simulink model "gm_sampleModel1541_4_sub_sub_sub"  (R2023a)
settings: Solver=VariableStepAuto  StartTime=0.0  StopTime=10.0  RelTol=1e-3
libraries: hdlsllib x4, simulink x3
settings Model: Creator=user1  LastModifiedBy=user1
settings OptimizationCC: BlockReduction=off  ConditionallyExecuteInputs=off
settings DebuggingCC: InheritedTsInSrcMsg=none

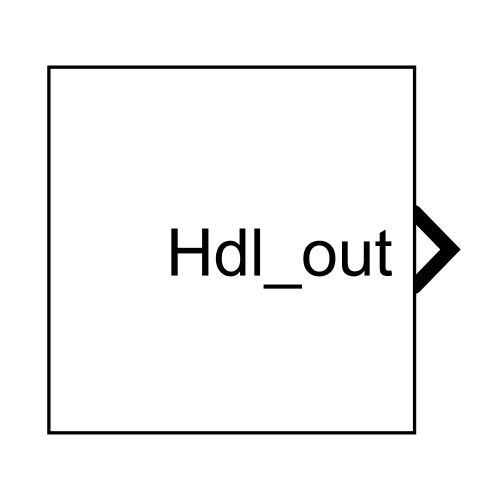
[thumbnail: Simulink's stored preview of the top-level diagram]
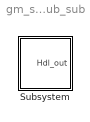
== system gm_sampleModel1541_4_sub_sub_sub ==
  Subsystem : Subsystem

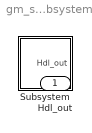
== system gm_sampleModel1541_4_sub_sub_sub/Subsystem ==
  Subsystem : Subsystem
  Hdl_out : Outport  OutDataTypeStr=uint8

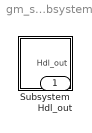
== system gm_sampleModel1541_4_sub_sub_sub/Subsystem/Subsystem ==
  Subsystem : Subsystem
  Hdl_out : Outport  OutDataTypeStr=uint8

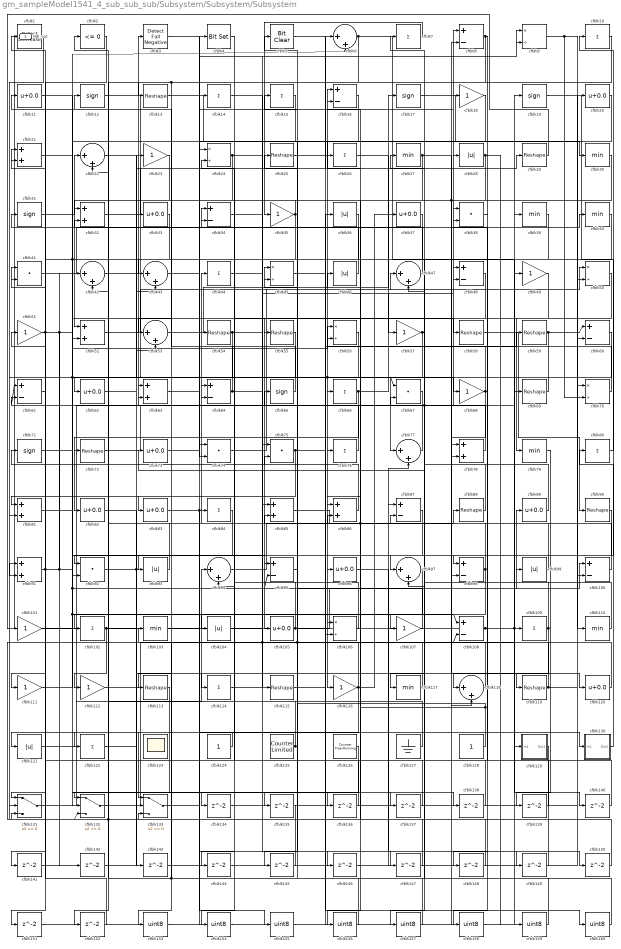
== system gm_sampleModel1541_4_sub_sub_sub/Subsystem/Subsystem/Subsystem ==
  cfblk1 : simulink/Logic and Bit Operations/Detect Decrease  vinit=0.0  OutDataTypeStr=uint8
      settings: LibrarySourceBlock=|
      | hdlsllib/Logic and Bit
      | Operations/Detect
      | Decrease
  cfblk{7,10,14..15,26,44,66,76,80,84,102,109,114,122} (14 alike) : Sum  Inputs=+  OutDataTypeStr=uint8
  cfblk{8,16,34,48,60..61,64,87,95,98,100,108} (12 alike) : Sum  Inputs=+-  OutDataTypeStr=uint8
  cfblk{18,23,35,49,51,57,68,101,107,111..112,116} (12 alike) : Gain  OutDataTypeStr=uint8
  cfblk{27,30,39..40,79,103,110,117} (8 alike) : MinMax  OutDataTypeStr=uint8
  cfblk{28,36,46,93,99,104,121} (7 alike) : Abs  OutDataTypeStr=uint8  SaturateOnIntegerOverflow=off
  cfblk{11,20,33,37,62,73,82..83,89,96,105,120} (12 alike) : Bias  Bias=0.0  SaturateOnIntegerOverflow=off
  cfblk{9,24,45,50,56,70,106} (7 alike) : Product  Inputs=*/  OutDataTypeStr=uint8  RndMeth=Zero  SaturateOnIntegerOverflow=on
  cfblk{13,25,29,54..55,58..59,69,72,88,90,113,115,119} (14 alike) : Reshape
  cfblk{6,22,42..43,47,53,77,94,97,118} (10 alike) : Sum  Inputs=|++  OutDataTypeStr=uint8
  cfblk{12,17,19,31,65,71} (6 alike) : Signum
  cfblk123 : Scope
      settings: Floating=on
  cfblk124 : Constant  OutDataTypeStr=uint8  SampleTime=-1
  cfblk125 : hdlsllib/Sources/Counter Limited  uplimit=7  tsamp=-1
  cfblk126 : hdlsllib/Sources/Counter Free-Running  NumBits=16  tsamp=-1
  cfblk127 : Ground
  cfblk128 : Constant  OutDataTypeStr=uint8  SampleTime=-1
  cfblk129 : Subsystem
      settings: LibrarySourceBlock=|
      | hdlsllib/Ports &
      | Subsystems/Subsystem
  cfblk130 : Subsystem
      settings: LibrarySourceBlock=|
      | hdlsllib/Ports &
      | Subsystems/Subsystem
  cfblk131 : Switch  OutDataTypeStr=uint8  SaturateOnIntegerOverflow=off  InputSameDT=off
  cfblk132 : Switch  OutDataTypeStr=uint8  SaturateOnIntegerOverflow=off  InputSameDT=off
  cfblk133 : Switch  OutDataTypeStr=uint8  SaturateOnIntegerOverflow=off  InputSameDT=off
  cfblk{134..152} (19 alike) : Delay  SampleTime=1
  cfblk{153..160} (8 alike) : DataTypeConversion  OutDataTypeStr=uint8  SaturateOnIntegerOverflow=off  RndMeth=Floor
  cfblk2 : hdlsllib/Logic and Bit Operations/Compare To Zero  relop=<=  OutDataTypeStr=uint8
  cfblk{21,32,52,63,78,81,85..86,91} (9 alike) : Sum  OutDataTypeStr=uint8
  cfblk3 : hdlsllib/Logic and Bit Operations/Detect Fall Negative  vinit=0  OutDataTypeStr=uint8
  cfblk{38,41,67,74..75,92} (6 alike) : DotProduct  OutDataTypeStr=uint8
  cfblk4 : simulink/Logic and Bit Operations/Bit Set  iBit=0
      settings: LibrarySourceBlock=|
      | hdlsllib/Logic and Bit
      | Operations/Bit Set
  cfblk5 : simulink/Logic and Bit Operations/Bit Clear  iBit=0
      settings: LibrarySourceBlock=|
      | hdlsllib/Logic and Bit
      | Operations/Bit Clear
  Hdl_out : Outport  OutDataTypeStr=uint8
  wires:
  cfblk160/1 -> cfblk97/2
  cfblk5/1 -> cfblk160/1
  cfblk159/1 -> cfblk5/1
  cfblk158/1 -> cfblk39/1
  cfblk157/1 -> cfblk132/3, cfblk12/1, cfblk133/3
  cfblk156/1 -> cfblk103/1
  cfblk30/1 -> cfblk156/1
  cfblk155/1 -> cfblk36/1
  cfblk103/1 -> cfblk155/1
  cfblk154/1 -> cfblk109/1
  cfblk4/1 -> cfblk154/1
  cfblk153/1 -> cfblk4/1
  cfblk152/1 -> cfblk41/2
  cfblk90/1 -> cfblk152/1
  cfblk151/1 -> cfblk118/2
  cfblk150/1 -> cfblk78/1
  cfblk44/1 -> cfblk150/1
  cfblk149/1 -> cfblk131/2
  cfblk96/1 -> cfblk149/1
  cfblk148/1 -> cfblk86/2
  cfblk147/1 -> cfblk74/1
  cfblk45/1 -> cfblk147/1
  cfblk146/1 -> cfblk8/2
  cfblk133/1 -> cfblk146/1
  cfblk145/1 -> cfblk91/1
  cfblk16/1 -> cfblk145/1
  cfblk144/1 -> cfblk100/2
  cfblk48/1 -> cfblk144/1
  cfblk143/1 -> cfblk77/2
  cfblk82/1 -> cfblk143/1
  cfblk142/1 -> cfblk70/1
  cfblk141/1 -> cfblk43/2
  cfblk140/1 -> cfblk38/2
  cfblk139/1 -> cfblk87/1
  cfblk79/1 -> cfblk139/1
  cfblk138/1 -> cfblk47/2
  cfblk137/1 -> cfblk1/1
  cfblk14/1 -> cfblk137/1
  cfblk136/1 -> cfblk64/2
  cfblk135/1 -> cfblk131/3
  cfblk60/1 -> cfblk135/1
  cfblk134/1 -> cfblk50/2
  cfblk97/1 -> cfblk134/1
  cfblk26/1 -> cfblk57/1
  cfblk33/1 -> cfblk81/1
  cfblk113/1 -> cfblk132/2
  cfblk46/1 -> cfblk24/2
  cfblk24/1 -> cfblk113/1, cfblk136/1
  cfblk100/1 -> cfblk26/1, cfblk42/2
  cfblk88/1 -> cfblk33/1, cfblk61/1
  cfblk20/1 -> cfblk92/2
  cfblk120/1 -> cfblk7/1
  cfblk81/1 -> cfblk106/1
  cfblk61/1 -> cfblk21/1
  cfblk127/1 -> cfblk22/2
  cfblk117/1 -> cfblk75/2
  cfblk114/1 -> cfblk46/1, cfblk108/2
  cfblk126/1 -> cfblk132/1
  cfblk89/1 -> cfblk31/1
  cfblk47/1 -> cfblk34/2
  cfblk10/1 -> cfblk13/1
  cfblk77/1 -> cfblk64/1
  cfblk1/1 -> cfblk91/2
  cfblk106/1 -> cfblk71/1
  cfblk116/1 -> cfblk45/1, cfblk37/1, cfblk133/1
  cfblk109/1 -> cfblk73/1, cfblk148/1
  cfblk107/1 -> cfblk25/1
  cfblk63/1 -> cfblk14/1
  cfblk95/1 -> cfblk65/1
  cfblk15/1 -> cfblk74/2
  cfblk9/1 -> cfblk60/2, cfblk70/2
  cfblk36/1 -> cfblk43/1
  cfblk13/1 -> cfblk75/1
  cfblk62/1 -> cfblk29/1
  cfblk87/1 -> cfblk92/1
  cfblk43/1 -> cfblk9/1
  cfblk132/1 -> cfblk69/1
  cfblk83/1 -> cfblk18/1, cfblk130/1(In1)
  cfblk68/1 -> cfblk16/2, cfblk98/2, cfblk158/1
  cfblk21/1 -> cfblk66/1, cfblk67/1, cfblk107/1
  cfblk128/1 -> cfblk85/2, cfblk56/2
  cfblk66/1 -> cfblk82/1, cfblk48/2
  cfblk85/1 -> cfblk87/2
  cfblk112/1 -> cfblk120/1
  cfblk72/1 -> cfblk19/1
  cfblk22/1 -> cfblk68/1
  cfblk91/1 -> cfblk95/1, cfblk42/1, cfblk41/1
  cfblk92/1 -> cfblk114/1, cfblk67/2
  cfblk59/1 -> cfblk60/1, cfblk81/2
  cfblk73/1 -> cfblk24/1
  cfblk98/1 -> cfblk122/1, cfblk27/1
  cfblk51/1 -> cfblk133/2, cfblk142/1, cfblk21/2
  cfblk111/1 -> cfblk6/2, cfblk95/2
  cfblk2/1 -> cfblk111/1
  cfblk130/1(Out1) -> cfblk80/1
  cfblk32/1 -> cfblk6/1
  cfblk11/1 -> cfblk55/1
  cfblk84/1 -> cfblk93/1
  cfblk101/1 -> cfblk56/1
  cfblk57/1 -> cfblk77/1, cfblk117/1
  cfblk31/1 -> cfblk22/1
  cfblk65/1 -> cfblk34/1
  cfblk55/1 -> cfblk131/1
  cfblk67/1 -> cfblk63/2
  cfblk8/1 -> cfblk102/1, cfblk83/1, cfblk98/1
  cfblk119/1 -> cfblk20/1, cfblk94/2
  cfblk40/1 -> cfblk104/1
  cfblk17/1 -> cfblk110/1
  cfblk115/1 -> cfblk59/1
  cfblk71/1 -> cfblk108/1, cfblk138/1
  cfblk86/1 -> cfblk54/1
  cfblk80/1 -> cfblk10/1
  cfblk125/1 -> cfblk84/1, cfblk45/2
  cfblk108/1 -> cfblk49/1, cfblk140/1, Hdl_out/1
  cfblk35/1 -> cfblk52/2, cfblk141/1, cfblk32/1
  cfblk122/1 -> cfblk23/1
  cfblk37/1 -> cfblk86/1
  cfblk23/1 -> cfblk52/1
  cfblk105/1 -> cfblk100/1, cfblk32/2
  cfblk93/1 -> cfblk2/1
  cfblk53/1 -> cfblk17/1
  cfblk129/1(Out1) -> cfblk51/1
  cfblk75/1 -> cfblk40/1, cfblk151/1
  cfblk121/1 -> cfblk94/1
  cfblk102/1 -> cfblk112/1, cfblk53/2
  cfblk12/1 -> cfblk115/1
  cfblk3/1 -> cfblk30/1
  cfblk76/1 -> cfblk63/1
  cfblk74/1 -> cfblk50/1
  cfblk29/1 -> cfblk101/1
  cfblk54/1 -> cfblk48/1, cfblk153/1
  cfblk58/1 -> cfblk90/1
  cfblk41/1 -> cfblk38/1
  cfblk38/1 -> cfblk118/1
  cfblk28/1 -> cfblk72/1, cfblk78/2, cfblk159/1
  cfblk6/1 -> cfblk129/1(In1), cfblk53/1
  cfblk42/1 -> cfblk58/1
  cfblk25/1 -> cfblk16/1
  cfblk64/1 -> cfblk11/1, cfblk9/2
  cfblk39/1 -> cfblk157/1
  cfblk118/1 -> cfblk15/1, cfblk61/2
  cfblk34/1 -> cfblk85/1
  cfblk49/1 -> cfblk79/1
  cfblk104/1 -> cfblk99/1
  cfblk131/1 -> cfblk28/1
  cfblk94/1 -> cfblk88/1
  cfblk78/1 -> cfblk3/1
  cfblk70/1 -> cfblk8/1
  cfblk7/1 -> cfblk35/1
  cfblk52/1 -> cfblk47/1
  cfblk56/1 -> cfblk76/1, cfblk106/2
  cfblk124/1 -> cfblk121/1
  cfblk18/1 -> cfblk96/1
  cfblk27/1 -> cfblk116/1, cfblk119/1
  cfblk99/1 -> cfblk44/1
  cfblk110/1 -> cfblk89/1
  cfblk69/1 -> cfblk62/1
  cfblk19/1 -> cfblk97/1
  cfblk50/1 -> cfblk105/1

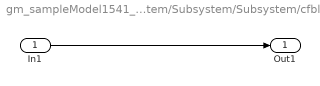
== system gm_sampleModel1541_4_sub_sub_sub/Subsystem/Subsystem/Subsystem/cfblk129 ==
  In1 : Inport
  Out1 : Outport
  wires:
  In1/1 -> Out1/1

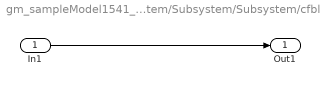
== system gm_sampleModel1541_4_sub_sub_sub/Subsystem/Subsystem/Subsystem/cfblk130 ==
  In1 : Inport
  Out1 : Outport
  wires:
  In1/1 -> Out1/1
